simulink model "PAN_rendezvous_GNC_block"  (R2017b)
settings: Solver=VariableStepAuto  StartTime=0.0  StopTime=10.0  RelTol=1e-3
undefined symbols (not defined in the file or in its folder): Imp_max, Imp_min, K_F, L_F, m_follower, match_tol, muE, ontime_max, ontime_min, Thrust_max, Thrust_min
libraries: hEemethod x8
settings Model: Creator=mtwal  LastModifiedBy=mtwal

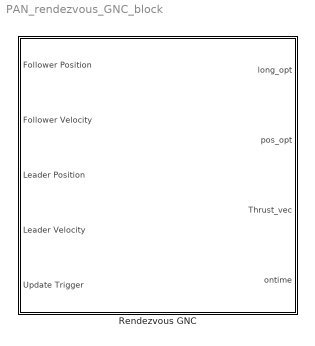
== system PAN_rendezvous_GNC_block ==
  Rendezvous GNC : Subsystem

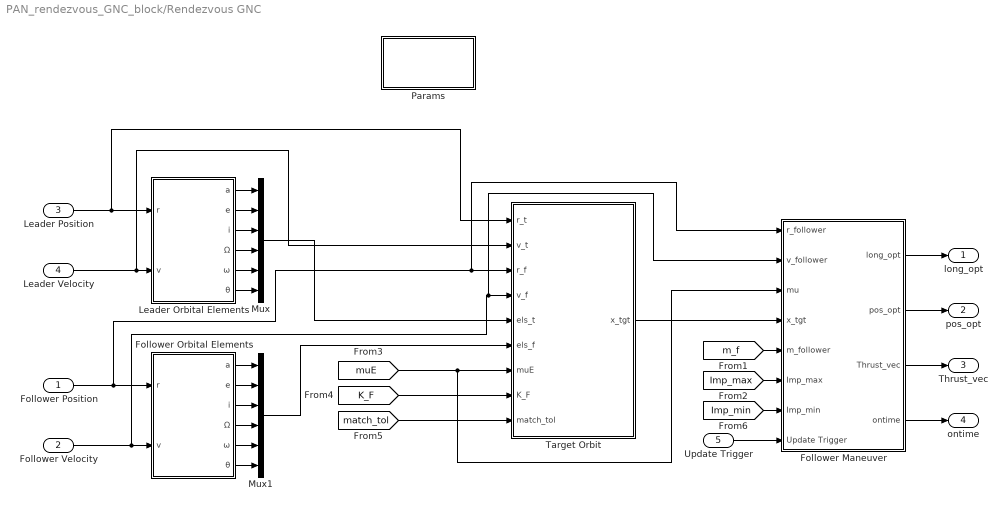
== system PAN_rendezvous_GNC_block/Rendezvous GNC ==
  Follower Position : Inport
  Follower Velocity : Inport  Port=2
  Leader Position : Inport  Port=3
  Leader Velocity : Inport  Port=4
  Update Trigger : Inport  Port=5
  Follower Maneuver : Subsystem
  Follower Orbital Elements : Subsystem
  Leader Orbital Elements : Subsystem
  Mux : Mux  Inputs=6
  Mux1 : Mux  Inputs=6
  Params : Subsystem
  Target Orbit : MATLAB Function  TreatAsAtomicUnit=on
  long_opt : Outport
  pos_opt : Outport  Port=2
  Thrust_vec : Outport  Port=3
  ontime : Outport  Port=4
  wires:
  [muE] -> Follower Maneuver/3(mu), Target Orbit/7(muE)
  [K_F] -> Target Orbit/8(K_F)
  [match_tol] -> Target Orbit/9(match_tol)
  Mux/1 -> Target Orbit/5(els_t)
  Leader Orbital Elements/5(ω) -> Mux/5
  Leader Velocity/1 -> Leader Orbital Elements/2(v), Target Orbit/2(v_t)
  Leader Position/1 -> Leader Orbital Elements/1(r), Target Orbit/1(r_t)
  Leader Orbital Elements/6(θ) -> Mux/6
  Leader Orbital Elements/2(e) -> Mux/2
  Leader Orbital Elements/3(i) -> Mux/3
  Leader Orbital Elements/1(a) -> Mux/1
  Leader Orbital Elements/4(Ω) -> Mux/4
  Mux1/1 -> Target Orbit/6(els_f)
  Follower Orbital Elements/5(ω) -> Mux1/5
  Follower Velocity/1 -> Follower Orbital Elements/2(v), Follower Maneuver/2(v_follower), Target Orbit/4(v_f)
  Follower Position/1 -> Follower Orbital Elements/1(r), Follower Maneuver/1(r_follower), Target Orbit/3(r_f)
  Follower Orbital Elements/6(θ) -> Mux1/6
  Follower Orbital Elements/2(e) -> Mux1/2
  Follower Orbital Elements/3(i) -> Mux1/3
  Follower Orbital Elements/1(a) -> Mux1/1
  Follower Orbital Elements/4(Ω) -> Mux1/4
  Target Orbit/1(x_tgt) -> Follower Maneuver/4(x_tgt)
  Update Trigger/1 -> Follower Maneuver/8(Update Trigger)
  Follower Maneuver/1(long_opt) -> long_opt/1
  Follower Maneuver/2(pos_opt) -> pos_opt/1
  Follower Maneuver/3(Thrust_vec) -> Thrust_vec/1
  Follower Maneuver/4(ontime) -> ontime/1
  [m_f] -> Follower Maneuver/5(m_follower)
  [Imp_max] -> Follower Maneuver/6(Imp_max)
  [Imp_min] -> Follower Maneuver/7(Imp_min)

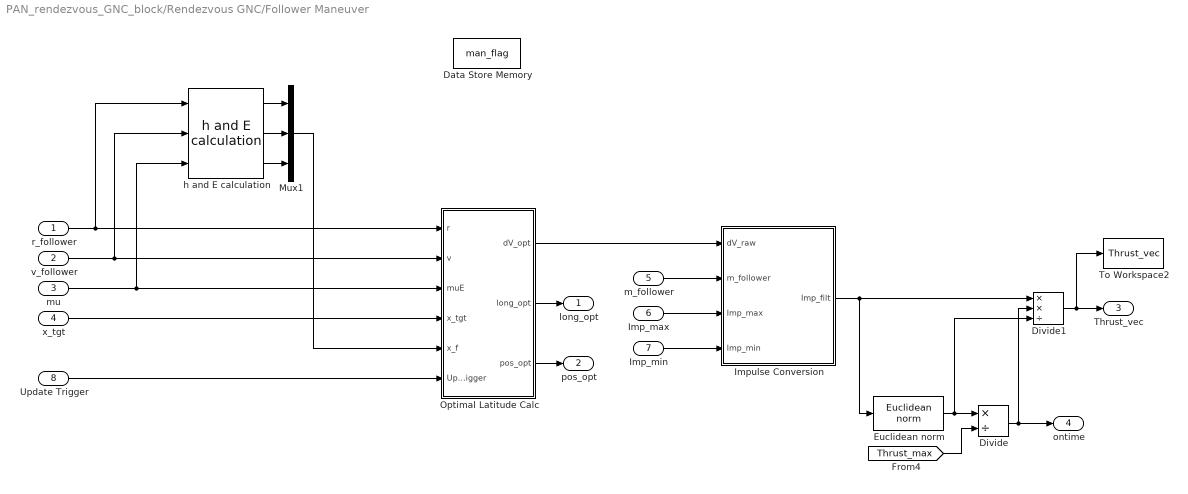
== system PAN_rendezvous_GNC_block/Rendezvous GNC/Follower Maneuver ==
  r_follower : Inport
  v_follower : Inport  Port=2
  mu : Inport  Port=3
  x_tgt : Inport  Port=4
  m_follower : Inport  Port=5
  Imp_max : Inport  Port=6
  Imp_min : Inport  Port=7
  Update Trigger : Inport  Port=8
  Data Store Memory : DataStoreMemory  DataStoreName=man_flag  WriteAfterWriteMsg=warning  WriteAfterReadMsg=warning  ShowAdditionalParam=off
  Divide : Product  Inputs=*/
  Divide1 : Product  Inputs=**/
  Euclidean norm : hEemethod/Math Operations/Euclidean norm
      settings: SourceProductName=HEe Method Library
  Impulse Conversion : MATLAB Function  TreatAsAtomicUnit=on
  Mux1 : Mux  Inputs=3
  Optimal Latitude Calc : Subsystem
  To Workspace2 : ToWorkspace  VariableName=Thrust_vec  SaveFormat=Timeseries  SampleTime=-1
  h and E calculation : hEemethod/Math Operations/h and E calculation
      settings: SourceProductName=HEe Method Library
  long_opt : Outport
  pos_opt : Outport  Port=2
  Thrust_vec : Outport  Port=3
  ontime : Outport  Port=4
  wires:
  r_follower/1 -> h and E calculation/1, Optimal Latitude Calc/1("r ")
  h and E calculation/1 -> Mux1/1
  h and E calculation/2 -> Mux1/2
  Mux1/1 -> Optimal Latitude Calc/5(x_f)
  x_tgt/1 -> Optimal Latitude Calc/4(x_tgt)
  mu/1 -> h and E calculation/3, Optimal Latitude Calc/3(muE)
  v_follower/1 -> h and E calculation/2, Optimal Latitude Calc/2("v ")
  h and E calculation/3 -> Mux1/3
  Optimal Latitude Calc/2(long_opt) -> long_opt/1
  Optimal Latitude Calc/1(dV_opt) -> Impulse Conversion/1(dV_raw)
  Imp_min/1 -> Impulse Conversion/4(Imp_min)
  Imp_max/1 -> Impulse Conversion/3(Imp_max)
  m_follower/1 -> Impulse Conversion/2(m_follower)
  Update Trigger/1 -> Optimal Latitude Calc/6(Update Trigger)
  Optimal Latitude Calc/3(pos_opt) -> pos_opt/1
  Euclidean norm/1 -> Divide1/3, Divide/1
  Divide1/1 -> To Workspace2/1, Thrust_vec/1
  [Thrust_max] -> Divide/2
  Divide/1 -> Divide1/2, ontime/1
  Impulse Conversion/1(Imp_filt) -> Euclidean norm/1, Divide1/1

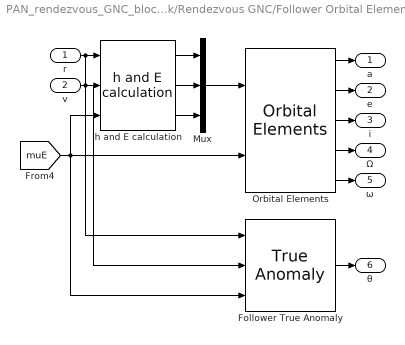
== system PAN_rendezvous_GNC_block/Rendezvous GNC/Follower Orbital Elements ==
  r : Inport
  v : Inport  Port=2
  Follower True Anomaly : hEemethod/Math Operations/True Anomaly
      settings: SourceProductName=HEe Method Library
  Mux : Mux  Inputs=3
  Orbital Elements : hEemethod/Math Operations/Orbital Elements
      settings: SourceProductName=HEe Method Library
  h and E calculation : hEemethod/Math Operations/h and E calculation
      settings: SourceProductName=HEe Method Library
  a : Outport
  e : Outport  Port=2
  i : Outport  Port=3
  Ω : Outport  Port=4
  ω : Outport  Port=5
  θ : Outport  Port=6
  wires:
  h and E calculation/1 -> Mux/1
  Orbital Elements/5 -> ω/1
  Orbital Elements/2 -> e/1
  Orbital Elements/3 -> i/1
  Orbital Elements/1 -> a/1
  r/1 -> Follower True Anomaly/1, h and E calculation/1
  Orbital Elements/4 -> Ω/1
  v/1 -> Follower True Anomaly/2, h and E calculation/2
  Mux/1 -> Orbital Elements/1
  h and E calculation/2 -> Mux/2
  h and E calculation/3 -> Mux/3
  [muE] -> Follower True Anomaly/3, Orbital Elements/2, h and E calculation/3
  Follower True Anomaly/1 -> θ/1

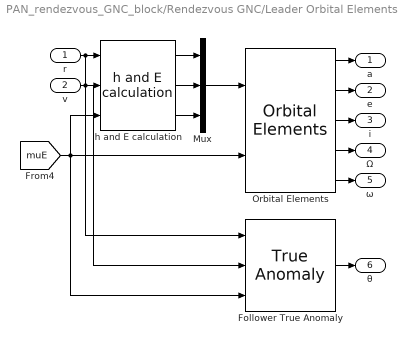
== system PAN_rendezvous_GNC_block/Rendezvous GNC/Leader Orbital Elements ==
  r : Inport
  v : Inport  Port=2
  Follower True Anomaly : hEemethod/Math Operations/True Anomaly
      settings: SourceProductName=HEe Method Library
  Mux : Mux  Inputs=3
  Orbital Elements : hEemethod/Math Operations/Orbital Elements
      settings: SourceProductName=HEe Method Library
  h and E calculation : hEemethod/Math Operations/h and E calculation
      settings: SourceProductName=HEe Method Library
  a : Outport
  e : Outport  Port=2
  i : Outport  Port=3
  Ω : Outport  Port=4
  ω : Outport  Port=5
  θ : Outport  Port=6
  wires:
  h and E calculation/1 -> Mux/1
  Orbital Elements/5 -> ω/1
  Orbital Elements/2 -> e/1
  Orbital Elements/3 -> i/1
  Orbital Elements/1 -> a/1
  r/1 -> Follower True Anomaly/1, h and E calculation/1
  Orbital Elements/4 -> Ω/1
  v/1 -> Follower True Anomaly/2, h and E calculation/2
  Mux/1 -> Orbital Elements/1
  h and E calculation/2 -> Mux/2
  h and E calculation/3 -> Mux/3
  [muE] -> Follower True Anomaly/3, Orbital Elements/2, h and E calculation/3
  Follower True Anomaly/1 -> θ/1

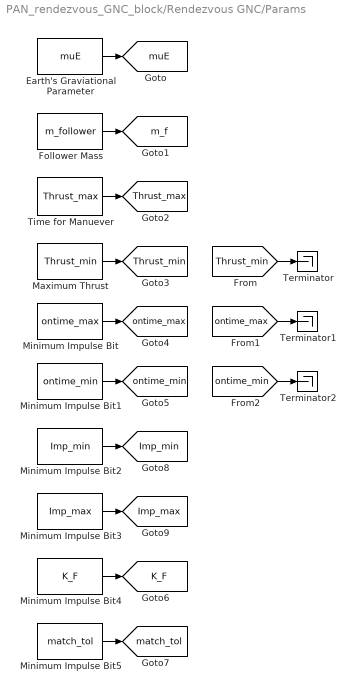
== system PAN_rendezvous_GNC_block/Rendezvous GNC/Params ==
  Earth's Graviational Parameter : Constant  Value=muE
  Follower Mass : Constant  Value=m_follower
  Maximum Thrust : Constant  Value=Thrust_min
  Minimum Impulse Bit : Constant  Value=ontime_max
  Minimum Impulse Bit1 : Constant  Value=ontime_min
  Minimum Impulse Bit2 : Constant  Value=Imp_min
  Minimum Impulse Bit3 : Constant  Value=Imp_max
  Minimum Impulse Bit4 : Constant  Value=K_F
  Minimum Impulse Bit5 : Constant  Value=match_tol
  Terminator : Terminator
  Terminator1 : Terminator
  Terminator2 : Terminator
  Time for Manuever : Constant  Value=Thrust_max
  tag scope: Imp_max=global, Imp_min=global, K_F=global, Thrust_max=global, Thrust_min=global, m_f=global, match_tol=global, muE=global, ontime_max=global, ontime_min=global
  wires:
  Time for Manuever/1 -> [Thrust_max]
  Follower Mass/1 -> [m_f]
  Earth's Graviational Parameter/1 -> [muE]
  Maximum Thrust/1 -> [Thrust_min]
  Minimum Impulse Bit/1 -> [ontime_max]
  Minimum Impulse Bit1/1 -> [ontime_min]
  Minimum Impulse Bit2/1 -> [Imp_min]
  Minimum Impulse Bit3/1 -> [Imp_max]
  [Thrust_min] -> Terminator/1
  [ontime_max] -> Terminator1/1
  [ontime_min] -> Terminator2/1
  Minimum Impulse Bit4/1 -> [K_F]
  Minimum Impulse Bit5/1 -> [match_tol]

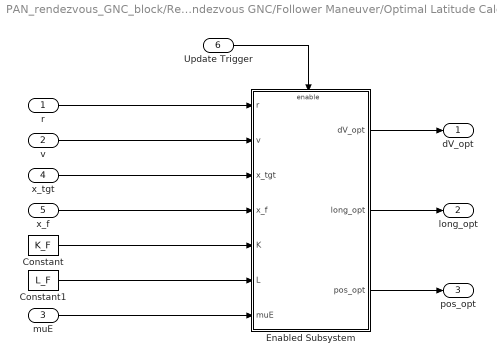
== system PAN_rendezvous_GNC_block/Rendezvous GNC/Follower Maneuver/Optimal Latitude Calc ==
  "r " : Inport
  "v " : Inport  Port=2
  muE : Inport  Port=3
  x_tgt : Inport  Port=4
  x_f : Inport  Port=5
  Update Trigger : Inport  Port=6
  Constant : Constant  Value=K_F
  Constant1 : Constant  Value=L_F
  Enabled Subsystem : Subsystem  TreatAsAtomicUnit=on
  dV_opt : Outport
  long_opt : Outport  Port=2
  pos_opt : Outport  Port=3
  wires:
  Enabled Subsystem/2(long_opt) -> long_opt/1
  "r "/1 -> Enabled Subsystem/1(r)
  "v "/1 -> Enabled Subsystem/2(v)
  muE/1 -> Enabled Subsystem/7("muE ")
  x_tgt/1 -> Enabled Subsystem/3(x_tgt)
  x_f/1 -> Enabled Subsystem/4(x_f)
  Constant/1 -> Enabled Subsystem/5(K)
  Constant1/1 -> Enabled Subsystem/6(L)
  Enabled Subsystem/1(dV_opt) -> dV_opt/1
  Enabled Subsystem/3(pos_opt) -> pos_opt/1
  Update Trigger/1 -> Enabled Subsystem/Enable

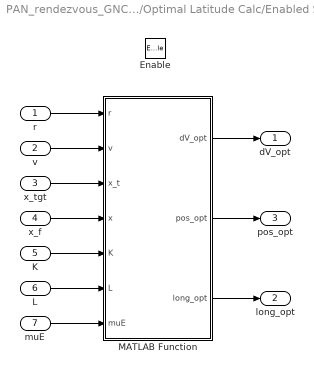
== system PAN_rendezvous_GNC_block/Rendezvous GNC/Follower Maneuver/Optimal Latitude Calc/Enabled Subsystem ==
  r : Inport
  v : Inport  Port=2
  x_tgt : Inport  Port=3
  x_f : Inport  Port=4
  K : Inport  Port=5
  L : Inport  Port=6
  "muE " : Inport  Port=7
  Enable : EnablePort
  MATLAB Function : MATLAB Function  TreatAsAtomicUnit=on
  dV_opt : Outport
  long_opt : Outport  Port=2
  pos_opt : Outport  Port=3
  wires:
  r/1 -> MATLAB Function/1(r)
  v/1 -> MATLAB Function/2(v)
  "muE "/1 -> MATLAB Function/7(muE)
  x_tgt/1 -> MATLAB Function/3(x_t)
  x_f/1 -> MATLAB Function/4(x)
  K/1 -> MATLAB Function/5(K)
  L/1 -> MATLAB Function/6(L)
  MATLAB Function/3(long_opt) -> long_opt/1
  MATLAB Function/1(dV_opt) -> dV_opt/1
  MATLAB Function/2(pos_opt) -> pos_opt/1

== matlab function PAN_rendezvous_GNC_block/Rendezvous GNC/Target Orbit ==
  data: r_t input; x_tgt output; v_t input; r_f input; v_f input; els_t input; els_f input; muE input; K_F input; match_tol input
function x_tgt = x_target(r_t,v_t,r_f,v_f,els_t,els_f,muE,K_F,match_tol)

h_f = cross(r_f,v_f);
E_f = -muE/(2*els_f(1));
ev_f = cross(v_f,h_f)/muE - r_f/norm(r_f);
x_f_current = [h_f;E_f;ev_f];

h_t = cross(r_t,v_t);
E_t = -muE/(2*els_t(1));
ev_t = cross(v_t,h_t)/muE - r_t/norm(r_t);
x_t_current = [h_t;E_t;ev_t];

if(~orb_matched(x_f_current,x_t_current,K_F,match_tol))
    x_tgt = x_t_current;
else
    pos_diff = r_t-r_f;
    vhat = v_f/norm(v_f);
    dr_vbar = dot(vhat,pos_diff)*vhat;
    along_track_sep = norm(dr_vbar);
    follower_ahead = (dot(vhat,pos_diff) < 0);

    if (norm(r_t-r_f) > 500000)
        if (follower_ahead)
            da_tgt = 500;
        else
            da_tgt = -500;
        end
    else
        [da_tgt,~] = decel_step(along_track_sep,follower_ahead);
    end

    a_tgt = els_t(1) + da_tgt;

    [~,~,x_tgt]=phasing_orbit(els_t,a_tgt,muE);
end

== matlab function PAN_rendezvous_GNC_block/Rendezvous GNC/Follower Maneuver/Optimal Latitude Calc/Enabled Subsystem/MATLAB Function ==
  data: dV_opt output; pos_opt output; long_opt output; r input; v input; x_t input; x input; K input; L input; muE input
function [dV_opt,pos_opt,long_opt] = fcn(r,v,x_t,x,K,L,muE)
%#codegen

z0=[r;v];

E=norm(v)^2/2-muE/norm(r);
a=-muE/(2*E);
T=2*pi/sqrt(muE)*a^(3/2);

options=odeset('AbsTol',1e-12,'RelTol',1e-12);
tspan=linspace(0,T,10000);
[~,zs] = ode45(@orbit1diff,tspan,z0,options,muE,[0;0;0]);

dV_opt = [0;0;0];
pos_opt = [0;0;0];
max_rat=0;
rat=0;
long_opt=0;
N=length(tspan);
x_f=x;
x_diff=x_t-x_f;
% x_diff_hat=x_diff/norm(x_diff);

for i=1:N
    r_f=zs(i,1:3);
    v_f=zs(i,4:6);
    
%     if (abs(dot(r_f,v_f))<perpTol)
%         rat=-999999;
%     end
    
    A=[crs(r_f);
       v_f];

    B=(crs(v_f)*crs(r_f)-crs(crs(r_f)*v_f'))/muE;    
    M=[A;
       B];

    dV_vec=pinv(M)*x_diff;
    dV_opt_sqd=dV_vec'*L*dV_vec;
    dx_vec=M*dV_vec;
    dx_opt_sqd=dx_vec'*K*dx_vec;
    
    rat=dx_opt_sqd/dV_opt_sqd;
    
    if (rat>max_rat)
        max_rat = rat;
        long_opt = atan2(r_f(2),r_f(1));
        pos_opt = r_f';
        dV_opt = dV_vec;
        if (long_opt<0)
            long_opt=long_opt+2*pi;
        end
    end
end
end

== matlab function PAN_rendezvous_GNC_block/Rendezvous GNC/Follower Maneuver/Impulse Conversion ==
  data: dV_raw input; m_follower input; Imp_filt output; Imp_max input; Imp_min input
function Imp_filt = fcn(dV_raw,m_follower,Imp_max,Imp_min)
%#codegen

Imp_raw = dV_raw*m_follower;

if (norm(Imp_raw)>Imp_max)
    Imp_red=Imp_raw*(Imp_max/norm(Imp_raw));
elseif (norm(Imp_raw)<Imp_min)
    Imp_red=[0;0;0];
else
    Imp_red=Imp_raw;
end

Imp_filt = Imp_red;
